simulink model "adaptive_adrc_controller"  (R2016a)
settings: Solver=ode45  StartTime=0.0  StopTime=100  RelTol=1e-3
model workspace (MAT data in the model file):
  k1 = 179.223891727
  k2 = 18.1352134536
settings Model: Creator=kbmaj  LastModifiedBy=kbmaj
settings DataIOCC: LimitDataPoints=on  SaveFormat=Array
settings HardwareCC: ProdBitPerPointer=32  ProdLargestAtomicFloat=None  ProdIntDivRoundTo=Undefined  ProdEndianess=Unspecified  ProdWordSize=32  ProdHWDeviceType=32-bit Generic
settings ModelReferenceCC: PropagateSignalLabelsOutOfModel=off
settings ConfigComp: CovModelRefEnable=Off

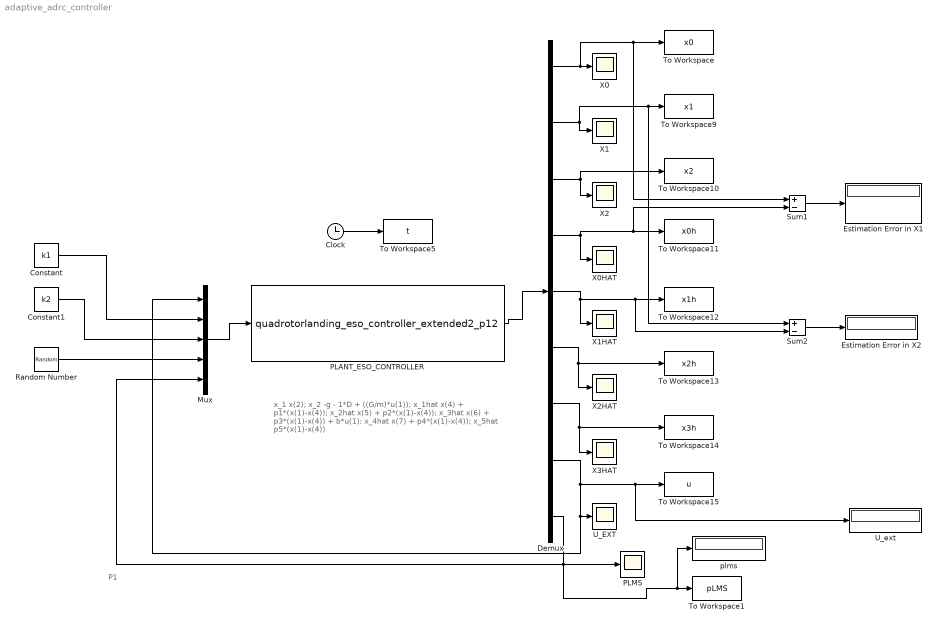
== system adaptive_adrc_controller ==
  note: P1
  note: x_1 x(2);
      | x_2 -g - 1*D + ((G/m)*u(1));
      | x_1hat x(4) + p1*(x(1)-x(4));
      | x_2hat x(5) + p2*(x(1)-x(4));
      | x_3hat x(6) + p3*(x(1)-x(4)) + b*u(1);
      | x_4hat x(7) + p4*(x(1)-x(4));
      | x_5hat p5*(x(1)-x(4))
  Clock : Clock
  Constant : Constant  Value=k1
  Constant1 : Constant  Value=k2
  Demux : Demux  Outputs=9
  Estimation Error in X1 : Display
  Estimation Error in X2 : Display
  Mux : Mux  Inputs=5
  PLANT_ESO_CONTROLLER : S-Function  FunctionName=quadrotorlanding_eso_controller_extended2_p12  SFunctionDeploymentMode=off  EnableBusSupport=off
  PLMS : Scope
  Random Number : RandomNumber  Variance=0  SampleTime=0
  Sum1 : Sum  Inputs=+-
  Sum2 : Sum  Inputs=+-
  To Workspace : ToWorkspace  VariableName=x0  SampleTime=-1
  To Workspace1 : ToWorkspace  VariableName=pLMS  SampleTime=-1
  To Workspace10 : ToWorkspace  VariableName=x2  SampleTime=-1
  To Workspace11 : ToWorkspace  VariableName=x0h  SampleTime=-1
  To Workspace12 : ToWorkspace  VariableName=x1h  SampleTime=-1
  To Workspace13 : ToWorkspace  VariableName=x2h  SampleTime=-1
  To Workspace14 : ToWorkspace  VariableName=x3h  SampleTime=-1
  To Workspace15 : ToWorkspace  VariableName=u  SampleTime=-1
  To Workspace5 : ToWorkspace  VariableName=t  SampleTime=-1
  To Workspace9 : ToWorkspace  VariableName=x1  SampleTime=-1
  U_EXT : Scope
  U_ext : Display
  X0 : Scope
  X0HAT : Scope
  X1 : Scope
  X1HAT : Scope
  X2 : Scope
  X2HAT : Scope
  X3HAT : Scope
  plms : Display
  wires:
  PLANT_ESO_CONTROLLER/1 -> Demux/1
  Constant/1 -> Mux/2
  Constant1/1 -> Mux/3
  Mux/1 -> PLANT_ESO_CONTROLLER/1
  Clock/1 -> To Workspace5/1
  Demux/1 -> To Workspace/1, Sum1/1, X0/1
  Demux/8 -> U_EXT/1, Mux/1, U_ext/1, To Workspace15/1
  Demux/2 -> X1/1, Sum2/1, To Workspace9/1
  Demux/3 -> X2/1, To Workspace10/1
  Demux/4 -> X0HAT/1, To Workspace11/1, Sum1/2
  Demux/5 -> X1HAT/1, Sum2/2, To Workspace12/1
  Demux/6 -> X2HAT/1, To Workspace13/1
  Demux/7 -> X3HAT/1, To Workspace14/1
  Sum1/1 -> Estimation Error in X1/1
  Sum2/1 -> Estimation Error in X2/1
  Random Number/1 -> Mux/4
  Demux/9 -> plms/1, To Workspace1/1, Mux/5, PLMS/1
